simulink model "model"  (R2023a)
settings: Solver=FixedStepAuto  StartTime=0.0  StopTime=inf  FixedStep=0.001  RelTol=1e-3
model workspace (MAT data in the model file):
  V = Simulink.Parameter
  V.Value = 0.1
  V.DataType = 'auto'
  V.DocUnits = 'm/s'
  V.Complexity = 'real'
  V.Dimensions = [1 1]
values from neighbouring files (symbols this model uses):
  V = getVariable(mdlWks, 'V')    [runMe.m]
libraries: simulink x1
settings Model: Creator=upattacini  LastModifiedBy=upattacini
settings DataIOCC: SignalLogging=off  DSMLogging=off  SaveTime=off  ReturnWorkspaceOutputs=off

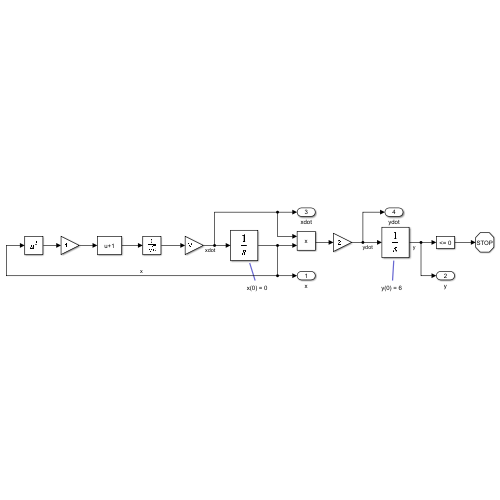
[thumbnail: Simulink's stored preview of the top-level diagram]
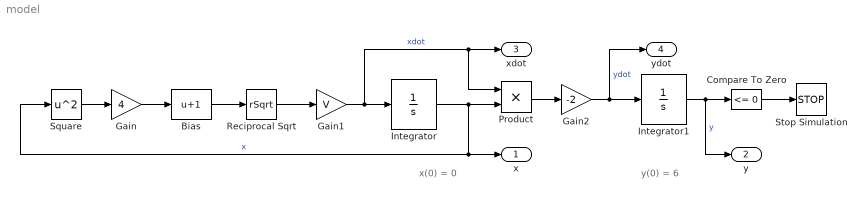
== system model ==
  note: y(0) = 6
  note: x(0) = 0
  Bias : Bias  Bias=1  SaturateOnIntegerOverflow=off
  Compare To Zero : simulink/Logic and Bit Operations/Compare To Zero  relop=<=  OutDataTypeStr=boolean
  Gain : Gain  Gain=4
  Gain1 : Gain  Gain=V
  Gain2 : Gain  Gain=-2
  Integrator : Integrator
  Integrator1 : Integrator  InitialCondition=6
  Product : Product
  Reciprocal Sqrt : Sqrt  Operator=rSqrt
  Square : Math  Operator=square
  Stop Simulation : Stop
  x : Outport
  y : Outport  Port=2
  xdot : Outport  Port=3
  ydot : Outport  Port=4
  wires:
  Square/1 -> Gain/1
  Gain/1 -> Bias/1
  Bias/1 -> Reciprocal Sqrt/1
  Reciprocal Sqrt/1 -> Gain1/1
  Gain1/1 -> Product/1, xdot/1, Integrator/1  "xdot"
  Integrator/1 -> Product/2, Square/1, x/1  "x"
  Compare To Zero/1 -> Stop Simulation/1
  Gain2/1 -> ydot/1, Integrator1/1  "ydot"
  Product/1 -> Gain2/1
  Integrator1/1 -> y/1, Compare To Zero/1  "y"
